simulink model "project_2_part2_ex3"  (R2026a)
settings: Solver=ode4  StopTime=Tfin  FixedStep=1e-3  MaxStep=1e-2  MinStep=1e-3  RelTol=5e-3
values from neighbouring files (symbols this model uses):
  refPoses = [Xr,Yr,psir]    [part2.m]
  zel = [Xl;Yl;psil;vxl;vyl;wpsil]    [part2.m]
settings Model: PacingRate=0.750000  Creator=The MathWorks, Inc.  LastModifiedBy=matte
settings SolverCC: ZeroCrossAlgorithm=Adaptive  DecoupledContinuousIntegration=on  MinimalZcImpactIntegration=on
settings DataIOCC: SaveFormat=StructureWithTime
settings OptimizationCC: BufferReuse=off
settings ConfigComp: PLC_TargetIDE=codesys35  PLC_MultiTBSigbuilderTimeRange=off  PLC_FoldFBCallOutputVar=off  PLC_RemoveUnusedSSMethodCallArguments=off  PLC_UseCallOutputArgSyntax=off  PLC_EnableUnsignedAndDoubleTypes=off  PLC_EnableUDTSplitting=off  PLC_MaxFieldsInUDT=500.0  PLC_InlineEnumCastFunction=off  PLC_RTWMaxIdLength=31.0  PLC_RollThreshold=5.0  PLC_ActiveTab=0.0  PLC_EnableStringLiteralTB=on  PLC_Enable64bitIntSupport=off

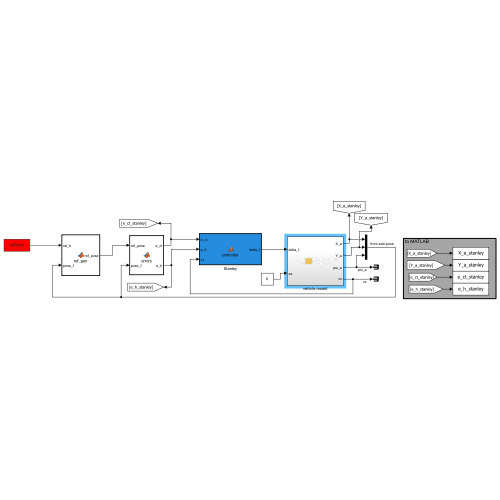
[thumbnail: Simulink's stored preview of the top-level diagram]
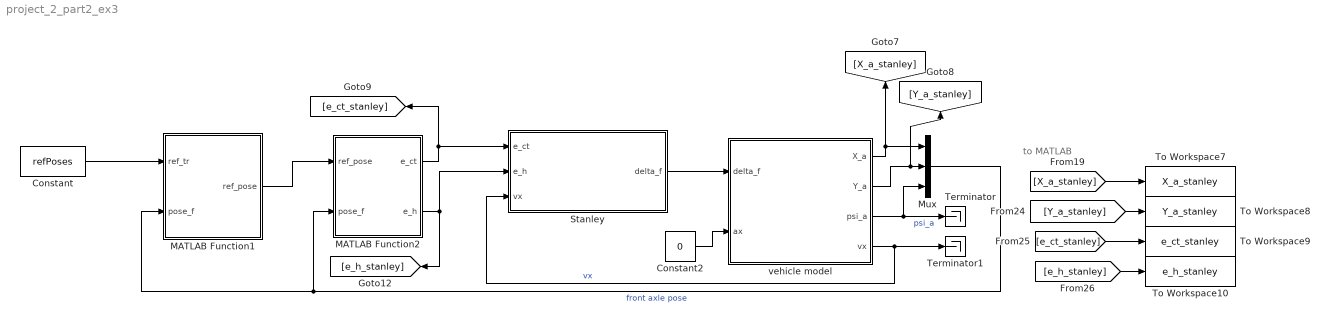
== system project_2_part2_ex3 ==
  note: to MATLAB
  Constant : Constant  Value=refPoses
  Constant2 : Constant  Value=0
  MATLAB Function1 : MATLAB Function  TreatAsAtomicUnit=on
  MATLAB Function2 : MATLAB Function  TreatAsAtomicUnit=on  VariantControl=Choice
  Mux : Mux  Inputs=3
  Stanley : MATLAB Function  TreatAsAtomicUnit=on
  Terminator : Terminator
  Terminator1 : Terminator
  To Workspace10 : ToWorkspace  VariableName=e_h_stanley  SaveFormat=Timeseries  SampleTime=-1
  To Workspace7 : ToWorkspace  VariableName=X_a_stanley  SaveFormat=Timeseries  SampleTime=-1
  To Workspace8 : ToWorkspace  VariableName=Y_a_stanley  SaveFormat=Timeseries  SampleTime=-1
  To Workspace9 : ToWorkspace  VariableName=e_ct_stanley  SaveFormat=Timeseries  SampleTime=-1
  vehicle model : Subsystem
  wires:
  Constant/1 -> MATLAB Function1/1(ref_tr)
  MATLAB Function1/1(ref_pose) -> MATLAB Function2/1(ref_pose)
  MATLAB Function2/2(e_h) -> Stanley/2(e_h), [e_h_stanley]
  Constant2/1 -> vehicle model/2(ax)
  Mux/1 -> MATLAB Function1/2(pose_f), MATLAB Function2/2(pose_f)  "front axle pose"
  vehicle model/1(X_a) -> Mux/1, [X_a_stanley]
  MATLAB Function2/1(e_ct) -> [e_ct_stanley], Stanley/1(e_ct)
  vehicle model/3(psi_a) -> Terminator/1, Mux/3  "psi_a"
  vehicle model/2(Y_a) -> Mux/2, [Y_a_stanley]
  vehicle model/4(vx) -> Terminator1/1, Stanley/3(vx)  "vx"
  [X_a_stanley] -> To Workspace7/1
  [Y_a_stanley] -> To Workspace8/1
  [e_ct_stanley] -> To Workspace9/1
  [e_h_stanley] -> To Workspace10/1
  Stanley/1(delta_f) -> vehicle model/1(delta_f)

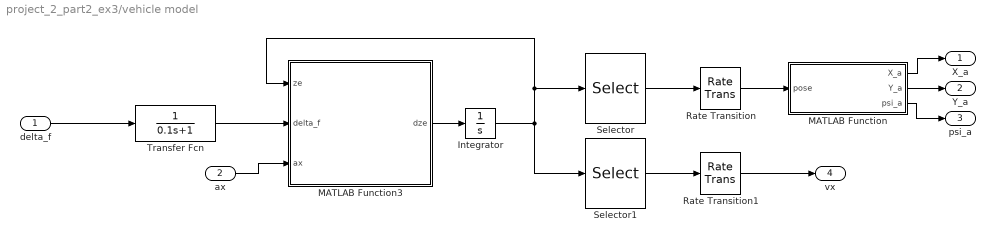
== system project_2_part2_ex3/vehicle model ==
  delta_f : Inport
  ax : Inport  Port=2
  Integrator : Integrator  InitialCondition=zel
  MATLAB Function : MATLAB Function  TreatAsAtomicUnit=on
  MATLAB Function3 : MATLAB Function  TreatAsAtomicUnit=on
  Rate Transition : RateTransition
  Rate Transition1 : RateTransition
  Selector : Selector  InputPortWidth=6  IndexOptions=Index vector (dialog)  Indices=[1:3]  OutputSizes=1
  Selector1 : Selector  InputPortWidth=6  IndexOptions=Index vector (dialog)  Indices=4  OutputSizes=1
  Transfer Fcn : TransferFcn  Denominator=[0.1 1]
  X_a : Outport
  Y_a : Outport  Port=2
  psi_a : Outport  Port=3
  vx : Outport  Port=4
  wires:
  ax/1 -> MATLAB Function3/3(ax)
  MATLAB Function3/1(dze) -> Integrator/1
  Integrator/1 -> MATLAB Function3/1(ze), Selector/1, Selector1/1
  Transfer Fcn/1 -> MATLAB Function3/2(delta_f)
  delta_f/1 -> Transfer Fcn/1
  Selector/1 -> Rate Transition/1
  MATLAB Function/1(X_a) -> X_a/1
  Rate Transition/1 -> MATLAB Function/1(pose)
  Selector1/1 -> Rate Transition1/1
  Rate Transition1/1 -> vx/1
  MATLAB Function/2(Y_a) -> Y_a/1
  MATLAB Function/3(psi_a) -> psi_a/1

== matlab function project_2_part2_ex3/MATLAB Function2 ==
  data: ref_pose input; e_ct output; pose_f input; e_h output
function [e_ct,e_h]=errors(ref_pose,pose_f)

% Wrap angles in the interval [0,2*pi]
ref_pose(3)=wrap_to_2pi(ref_pose(3));
pose_f(3)=wrap_to_2pi(pose_f(3));

% Cross-track error  
d=ref_pose(1:2)-pose_f(1:2);
e_ct=d(2)*cos(ref_pose(3))-d(1)*sin(ref_pose(3));

% Heading error
e_h=wrap_to_pi(ref_pose(3)-pose_f(3));

end

%--------------------------------------------------------------------------

function lambda = wrap_to_2pi(lambda)
%   Wraps angle in radians to [0 2*pi]
%   lambdaWrapped = wrapTo2Pi(LAMBDA) wraps angles in LAMBDA, in radians,
%   to the interval [0 2*pi] such that zero maps to zero and 2*pi maps
%   to 2*pi. (In general, positive multiples of 2*pi map to 2*pi and
%   negative multiples of 2*pi map to zero.)
%   See also wrapToPi, wrapTo180, wrapTo360.
positiveInput = (lambda > 0);
lambda = mod(lambda, 2*pi);
lambda((lambda == 0) & positiveInput) = 2*pi;
end

function lambda = wrap_to_pi(lambda)
%   Wraps angle in radians to [-pi pi]
%   lambdaWrapped = wrapToPi(LAMBDA) wraps angles in LAMBDA, in radians,
%   to the interval [-pi pi] such that pi maps to pi and -pi maps to
%   -pi.  (In general, odd, positive multiples of pi map to pi and odd,
%   negative multiples of pi map to -pi.)
%   See also wrapTo2Pi, wrapTo180, wrapTo360.
q = (lambda < -pi) | (pi < lambda);
lambda(q) = wrap_to_2pi(lambda(q) + pi) - pi;
end

== matlab function project_2_part2_ex3/MATLAB Function1 ==
  data: ref_tr input; ref_pose output; pose_f input
function ref_pose=ref_gen(ref_tr,pose_f)

N=size(ref_tr,1);

% reference trajectory closest point to the vehicle
dis=vecnorm(ref_tr(:,1:2)'-pose_f(1:2)*ones(1,N));
[~,c]=min(dis);
ref_pose=ref_tr(c,:)';

end

== matlab function project_2_part2_ex3/vehicle model/MATLAB Function3 ==
  data: ze input; delta_f input; dze output; ax input
function dze = DSTP_nonlinear_model(ze,delta_f, ax)

% States
X = ze(1);
Y =ze(2);
psi = ze(3);
vx = ze(4);
vy = ze(5);
wpsi = ze(6);

% % Inputs
% ax    = u(1);
% delta_f = u(2);

% Vehicle parameters:
l1 = 1.2;       % m
l2 = 1.6;       % m
m = 1575;       % kg
Jz = 4000;      % kg*m^2
C1 = 27e3;      % N/rad
C2 = C1;

% Slip angles (non-linear model)
alpha1 = atan((vy + l1*wpsi)/vx) - delta_f;
alpha2 = atan((vy - l2*wpsi)/vx);

% Pacejka's tire model
[fp_alpha1, fp_alpha2] = pacejka_model(alpha1,alpha2,C1,C2);
Fy1 = -fp_alpha1 * cos(delta_f);
Fy2 = -fp_alpha2;

% State equations
dX    = vx*cos(psi) - vy*sin(psi);
dY    = vx*sin(psi) + vy*cos(psi);
dpsi  = wpsi;
dvx   = vy*wpsi + ax;
dvy   = -vx*wpsi + (2/m)*(Fy1 + Fy2);
dwpsi = (2/Jz)*(l1*Fy1 - l2*Fy2);

dze = [dX; dY; dpsi; dvx; dvy; dwpsi];

% Pacejka Lateral tire forces 
function [fp_alpha1, fp_alpha2] = pacejka_model(alpha1,alpha2,C1,C2)

% Tire parameters:
p1 = 3863;      % N
p2 = 1.5;
p4 = -0.5;
p3_front = C1/p1/p2;  % front tire
p3_rear = C2/p1/p2;   % rear tire

fp_alpha1 = p1*sin(p2*atan(p3_front*alpha1 - p4*(p3_front*alpha1 - atan(p3_front*alpha1))));
fp_alpha2 = p1*sin(p2*atan(p3_rear*alpha2 - p4*(p3_rear*alpha2 - atan(p3_rear*alpha2))));

end
end

== matlab function project_2_part2_ex3/vehicle model/MATLAB Function ==
  data: pose input; X_a output; Y_a output; psi_a output
function [X_a,Y_a,psi_a] = translatePose(pose)
% Parameters
l1 = 1.2;       % m
X_CoG = pose(1);
Y_CoG = pose(2);
psi = pose(3);

% Front axle position
X_a = X_CoG + l1*cos(psi);
Y_a = Y_CoG + l1*sin(psi);
psi_a = psi;
end

== matlab function project_2_part2_ex3/Stanley ==
  data: e_ct input; delta_f output; e_h input; vx input
function delta_f = controller(e_ct,e_h,vx)
% % Stanley's parameters
Ks = 0.6;
v_b = 1;
delta_max = 35;     % deg

delta_f = e_h + atan((Ks*e_ct) / (v_b + vx));

% % Saturation of delta_f
if delta_f >= delta_max
    delta_f = delta_max;
    
elseif delta_f < -delta_max || delta_f > delta_max
    delta_f = delta_f;

elseif delta_f <= -delta_max
    delta_f = -delta_max;
end

end
